simulink model "Simulation_wrapped_4"  (R2015a)
settings: Solver=ode4  SolverMode=SingleTasking  StartTime=0.0  StopTime=20  FixedStep=0.001  MaxStep=0.01  RelTol=1e-3
InitFcn:
  | gen_signal
  | Read_aero_spreadsheet
  | model_params3
undefined symbols (not defined in the file or in its folder): acm_aero_model, acm_pitch_deg_ini, acm_pitch_rate_deg_s_ini, acm_T_N, breakpoints1, Cm0, Cmde, Cmq, dail, de, dele, drud, Fr_mp_1, Fr_mp_2, Fr_rp_1, Fr_rp_2, ini_acm_de_deg, ini_acm_p_deg_per_s, ini_acm_phi_deg, ini_acm_psi_deg, ini_acm_q_deg_per_s, ini_acm_r_deg_per_s, ini_acm_theta_deg, ini_cmp_de_deg, ini_rig_p_deg_per_s, ini_rig_phi_deg, ini_rig_psi_deg, ini_rig_q_deg_per_s, ini_rig_r_deg_per_s, ini_rig_theta_deg, ini_rig_theta_deg_per_s, K1_svo_acm, K1_svo_cmp, K2_svo_acm, K2_svo_cmp, K_de_nz2, K_de_q2, K_de_tht2, La, Ma, max_defl_sat_acm, max_defl_sat_cmp, max_rate_sat, max_rate_sat_acm, max_rate_sat_cmp, Na, rig_pitch_deg_ini, rig_pitch_rate_deg_s_ini, sigbuilder_block, simstop, windspeed, Xa, Ya, Za
libraries: aerolibconvert2 x96, simulink x40, aerolibtransform2 x18, vrlib x7
(part 1 of 6)
settings Model: CovSFcnEnable=off  Creator=PD Banneheka  LastModifiedBy=PD Banneheka
settings DataIOCC: SignalLoggingSaveFormat=ModelDataLogs  ReturnWorkspaceOutputs=on
settings DebuggingCC: ReadBeforeWriteMsg=DisableAll  WriteAfterWriteMsg=DisableAll  WriteAfterReadMsg=DisableAll  AlgebraicLoopMsg=none  ArtificialAlgebraicLoopMsg=none  UnderspecifiedInitializationDetection=Classic  MergeDetectMultiDrivingBlocksExec=none  SolverPrmCheckMsg=warning  MultiTaskDSMMsg=warning  MultiTaskCondExecSysMsg=none  StateNameClashWarn=warning
settings HardwareCC: ProdBitPerInt=16  ProdBitPerPointer=16  ProdWordSize=16  ProdHWDeviceType=Generic->16-bit Embedded Processor
settings ModelReferenceCC: UpdateModelReferenceTargets=IfOutOfDate  ModelReferenceMinAlgLoopOccurrences=on
settings SFSimCC: SimUserIncludeDirs=D:\PhD\2016\Week_27_25_Apr\Matlab\Simulation_load_cell\HHIRM  SFSimEcho=off

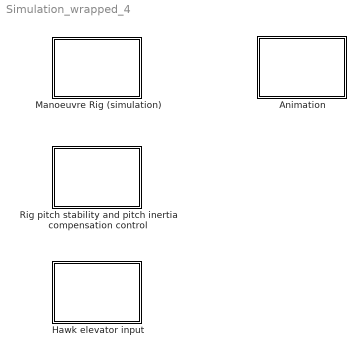
== system Simulation_wrapped_4 ==
  Animation : Subsystem
  Hawk elevator input : Subsystem
  Manoeuvre Rig (simulation) : Subsystem
  "Rig pitch stability and pitch inertia compensation control " : Subsystem

== system Simulation_wrapped_4/Animation ==
  Rotation Matrix to VRML Rotation{,1,3..6} (6 alike) : vrlib/Utilities/Rotation Matrix to VRML Rotation  maxzero=1e-12
  VR Sink : vrlib/VR Sink  InstantiateOnLoad=on  SampleTime=-1  ViewEnable=on  RemoteChange=off  RemoteView=off  FieldsWritten=Compensator.rotation.4.1.1.double#Compensator.translation.3.1.1.double#Arm.rotation.4.1.1.double#Arm.translation.3.1.1.double#Aircraft_model.rotation.4.1.1.double#Aircraft_model.translation.3.1.1.double#Back_added_mass.rotation.4.1.1.double#Back_added_mass.translation.3.1.1.double#Load_cell.rotation.4.1.1.double#Load_cell.translation.3.1.1.double#Link.rotation.4.1.1.double#Link.translation.3.1.1.double  WorldFileName=Animation.wrl  AutoView=on  VideoDimensions=[]  AllowVariableSize=off  FigureProperties="{'Position', 'Name', 'Viewpoint', 'CameraBound', 'CameraDirection', 'CameraPosition', 'CameraUpVector', 'ZoomFactor', 'Antialiasing', 'Headlight', 'Lighting', 'NavPanel', 'Sound', 'StatusBar', 'Stereo3D', 'Stereo3DCameraOffset', 'Stereo3DHIT', 'ToolBar', 'Textures', 'Transparency', 'Triad', 'Wireframe', 'NavZones', 'NavMode', 'NavSpeed', 'CaptureFileFormat', 'CaptureFileName', 'Record2DCompressMethod', 'Record2DCompressQuality', 'Record2D', 'Record2DFileName', 'Record2DFPS'; [1.9220000000000000e+03   8.4000000000000000e+01   9.5800000000000000e+02   3.8400000000000000e+02], '', 'Side view', 'on', [0.0000000000000000e+00   0.0000000000000000e+00  -1.0000000000000000e+00], [0.0000000000000000e+00   0.0000000000000000e+00   0.0000000000000000e+00], [0.0000000000000000e+00   1.0000000000000000e+00   0.0000000000000000e+00], [1.0000000000000000e+00], 'on', 'on', 'on', 'halfbar', 'on', 'on', 'off', [1.0000000149011612e-01], [0.0000000000000000e+00], 'on', 'on', 'on', 'none', 'off', 'off', 'fly', 'normal', 'tif', '%f_anim_%n.tif', 'auto', [7.5000000000000000e+01], 'off', '%f_anim_%n.avi', 'auto'}"
  wires:
  [animation_cmp_rotation] -> Rotation Matrix to VRML Rotation/1
  [animation_acm_rotation] -> Rotation Matrix to VRML Rotation4/1
  [animation_mass_rotation] -> Rotation Matrix to VRML Rotation3/1
  [animation_arm_rotation] -> Rotation Matrix to VRML Rotation1/1
  [animation_load_cell_rotation] -> Rotation Matrix to VRML Rotation5/1
  [animation_link_rotation] -> Rotation Matrix to VRML Rotation6/1
  [animation_link_translation] -> VR Sink/12
  Rotation Matrix to VRML Rotation/1 -> VR Sink/1
  [animation_cmp_translation] -> VR Sink/2
  Rotation Matrix to VRML Rotation1/1 -> VR Sink/3
  [animation_arm_translation] -> VR Sink/4
  Rotation Matrix to VRML Rotation4/1 -> VR Sink/5
  [animation_acm_translation] -> VR Sink/6
  Rotation Matrix to VRML Rotation3/1 -> VR Sink/7
  [animation_mass_translation] -> VR Sink/8
  Rotation Matrix to VRML Rotation5/1 -> VR Sink/9
  [animation_load_cell_translation] -> VR Sink/10
  Rotation Matrix to VRML Rotation6/1 -> VR Sink/11

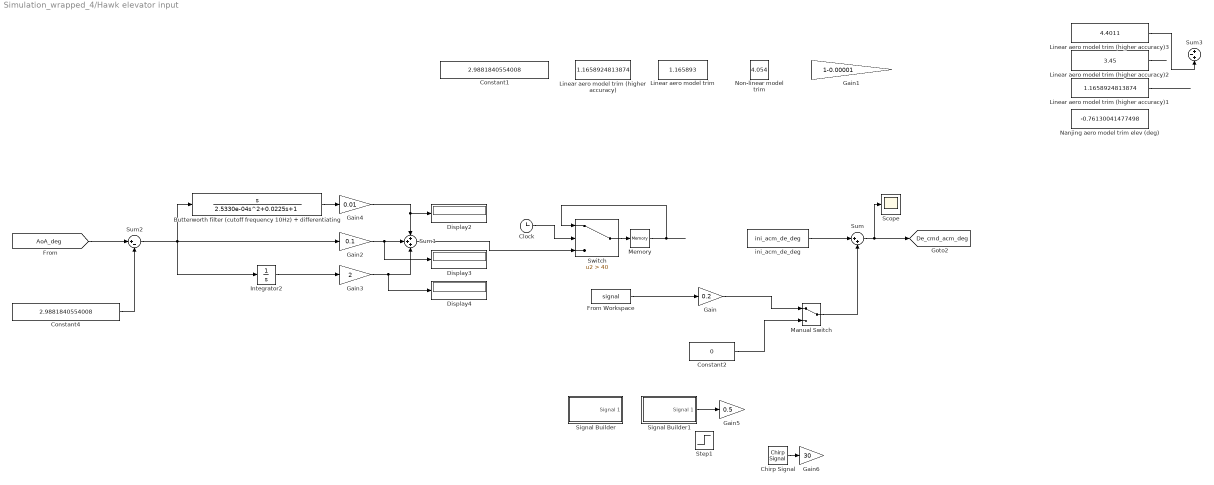
== system Simulation_wrapped_4/Hawk elevator input ==
  Butterworth filter (cutoff frequency 10Hz) + differentiating : TransferFcn  Numerator=[1 0]  Denominator=[2.5330e-04 0.0225 1]
  Chirp Signal : simulink/Sources/Chirp Signal  f1=0.1  T=100  f2=1
  Clock : Clock
  Constant1 : Constant  Value=2.9881840554008
  Constant2 : Constant  Value=0
  Constant4 : Constant  Value=2.9881840554008
  Display2 : Display
  Display3 : Display
  Display4 : Display
  From Workspace : FromWorkspace  VariableName=signal  SampleTime=0  OutputAfterFinalValue=Setting to zero
  Gain : Gain  Gain=0.2
  Gain1 : Gain  Gain=1-0.00001
  Gain2 : Gain  Gain=0.1
  Gain3 : Gain  Gain=2
  Gain4 : Gain  Gain=0.01
  Gain5 : Gain  Gain=0.5
  Gain6 : Gain  Gain=30
  Integrator2 : Integrator
  Linear aero model trim : Constant  Value=1.165893
  Linear aero model trim (higher accuracy) : Constant  Value=1.1658924813874
  Linear aero model trim (higher accuracy)1 : Constant  Value=1.1658924813874
  Linear aero model trim (higher accuracy)2 : Constant  Value=3.45
  Linear aero model trim (higher accuracy)3 : Constant  Value=4.4011
  Manual Switch : ManualSwitch
  Memory : Memory
  Nanjing aero model trim elev (deg) : Constant  Value=-0.76130041477498
  Non-linear model trim : Constant  Value=4.054
  Scope : Scope
      settings: SaveName=ScopeData7
  Signal Builder : Subsystem  Tag=STV Subsys  LoadFcn=sigbuilder_block('load');  StartFcn=sigbuilder_block('start');  StopFcn=sigbuilder_block('stop');  ClipboardFcn=sigbuilder_block('clipboard');  mask(Sigbuilder block){}
      mask help: Simulink:masks:SigbuilderBlock_MD
      mask init:
      | if ~strcmp(get_param(bdroot(gcbh),'SimulationStatus'),'stopped') tuvar = sigbuilder_block('maskInit'); end
      settings: CopyFcn=sigbuilder_block('copy');  DeleteFcn=sigbuilder_block('delete');  ModelCloseFcn=sigbuilder_block('modelClose');  PreSaveFcn=sigbuilder_block('preSave');  PauseFcn=sigbuilder_block('pause');  ContinueFcn=sigbuilder_block('continue');  NameChangeFcn=sigbuilder_block('namechange');  OpenFcn=sigbuilder_block('open',[437.6 199.2 550.4 400 ]);  CloseFcn=sigbuilder_block('close');
      mask Display: plot(0, 0, 100, 100,[2, 2, 32, 32, 2], [68, 8, 8, 68, 68],[32, 2], [38, 38], [32, 19, 2],[53, 60, 44], [32, 17, 17, 2],[16, 16, 31, 31]);txt = getActiveGroup(gcbh);text(2, 100, txt,'verticalAlignment', 'top');
  Signal Builder1 : Subsystem  Tag=STV Subsys  LoadFcn=sigbuilder_block('load');  StartFcn=sigbuilder_block('start');  StopFcn=sigbuilder_block('stop');  ClipboardFcn=sigbuilder_block('clipboard');  mask(Sigbuilder block){}
      mask help: Simulink:masks:SigbuilderBlock_MD
      mask init:
      | if ~strcmp(get_param(bdroot(gcbh),'SimulationStatus'),'stopped') tuvar = sigbuilder_block('maskInit'); end
      settings: CopyFcn=sigbuilder_block('copy');  DeleteFcn=sigbuilder_block('delete');  ModelCloseFcn=sigbuilder_block('modelClose');  PreSaveFcn=sigbuilder_block('preSave');  PauseFcn=sigbuilder_block('pause');  ContinueFcn=sigbuilder_block('continue');  NameChangeFcn=sigbuilder_block('namechange');  OpenFcn=sigbuilder_block('open',[437.6 199.2 550.4 400 ]);  CloseFcn=sigbuilder_block('close');
      mask Display: plot(0, 0, 100, 100,[2, 2, 32, 32, 2], [68, 8, 8, 68, 68],[32, 2], [38, 38], [32, 19, 2],[53, 60, 44], [32, 17, 17, 2],[16, 16, 31, 31]);txt = getActiveGroup(gcbh);text(2, 100, txt,'verticalAlignment', 'top');
  Step1 : Step  After=40-4.4011  SampleTime=0
  Sum : Sum  Inputs=|++
  Sum1 : Sum  Inputs=+++
  Sum2 : Sum  Inputs=|+-
  Sum3 : Sum  Inputs=+-+
  Switch : Switch  Criteria=u2 > Threshold  Threshold=40
  ini_acm_de_deg : Constant  Value=ini_acm_de_deg
  tag scope: De_cmd_acm_deg=global
  wires:
  From Workspace/1 -> Gain/1
  Manual Switch/1 -> Sum/2
  Gain/1 -> Manual Switch/1
  Integrator2/1 -> Gain3/1
  Sum2/1 -> Integrator2/1, Gain2/1, Butterworth filter (cutoff frequency 10Hz) + differentiating/1
  Butterworth filter (cutoff frequency 10Hz) + differentiating/1 -> Gain4/1
  Gain2/1 -> Display3/1, Sum1/2
  Gain4/1 -> Display2/1, Sum1/1
  Gain3/1 -> Display4/1, Sum1/3
  Sum1/1 -> Switch/3
  Switch/1 -> Memory/1
  Clock/1 -> Switch/2
  Memory/1 -> Switch/1
  [AoA_deg] -> Sum2/1
  Constant4/1 -> Sum2/2
  ini_acm_de_deg/1 -> Sum/1
  Signal Builder1/1(Signal 1) -> Gain5/1
  Sum/1 -> Scope/1, [De_cmd_acm_deg]
  Constant2/1 -> Manual Switch/2
  Chirp Signal/1 -> Gain6/1
  Linear aero model trim (higher accuracy)3/1 -> Sum3/3
  Linear aero model trim (higher accuracy)1/1 -> ?
  Linear aero model trim (higher accuracy)2/1 -> ?

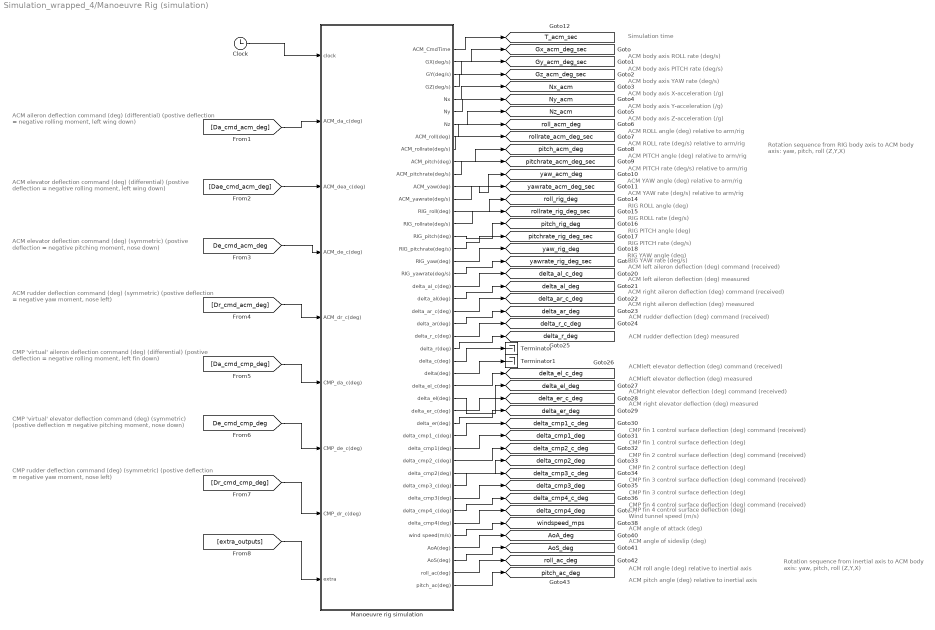
== system Simulation_wrapped_4/Manoeuvre Rig (simulation) ==
  note: ACM aileron deflection command (deg) (differential)
      | (postive deflection = negative rolling moment, left wing down)
  note: Wind tunnel speed (m/s)
  note: CMP fin 1 control surface deflection (deg) command (received)
  note: ACM left aileron deflection (deg) command (received)
  note: Simulation time
  note: ACM body axis ROLL rate (deg/s)
  note: ACM body axis PITCH rate (deg/s)
  note: ACM body axis YAW rate (deg/s)
  note: ACM body axis X-acceleration (/g)
  note: ACM body axis Y-acceleration (/g)
  note: ACM body axis Z-acceleration (/g)
  note: ACM ROLL angle (deg) relative to arm/rig
  note: ACM PITCH angle (deg) relative to arm/rig
  note: ACM YAW angle (deg) relative to arm/rig
  note: Rotation sequence from RIG body axis to ACM
      | body axis: yaw, pitch, roll (Z,Y,X)
  note: ACM ROLL rate (deg/s) relative to arm/rig
  note: ACM PITCH rate (deg/s) relative to arm/rig
  note: ACM YAW rate (deg/s) relative to arm/rig
  note: RIG ROLL angle (deg)
  note: RIG PITCH angle (deg)
  note: RIG YAW angle (deg)
  note: RIG ROLL rate (deg/s)
  note: RIG PITCH rate (deg/s)
  note: RIG YAW rate (deg/s)
  note: ACM left aileron deflection (deg) measured
  note: ACM right aileron deflection (deg) measured
  note: ACM right aileron deflection (deg) command (received)
  note: ACM rudder deflection (deg) measured
  note: ACM rudder deflection (deg) command (received)
  note: ACMleft elevator deflection (deg) measured
  note: ACMleft elevator deflection (deg) command (received)
  note: ACM right elevator deflection (deg) measured
  note: ACMright elevator deflection (deg) command (received)
  note: CMP fin 1 control surface deflection (deg)
  note: CMP fin 2 control surface deflection (deg) command (received)
  note: CMP fin 2 control surface deflection (deg)
  note: CMP fin 3 control surface deflection (deg) command (received)
  note: CMP fin 3 control surface deflection (deg)
  note: CMP fin 4 control surface deflection (deg) command (received)
  note: CMP fin 4 control surface deflection (deg)
  note: ACM angle of attack (deg)
  note: ACM angle of sideslip (deg)
  note: ACM roll angle (deg) relative to inertial axis
  note: ACM pitch angle (deg) relative to inertial axis
  note: Rotation sequence from inertial axis to ACM
      | body axis: yaw, pitch, roll (Z,Y,X)
  note: ACM elevator deflection command (deg) (symmetric)
      | (postive deflection = negative pitching moment, nose down)
  note: ACM rudder deflection command (deg) (symmetric)
      | (postive deflection = negative yaw moment, nose left)
  note: CMP 'virtual' aileron deflection command (deg) (differential)
      | (postive deflection = negative rolling moment, left fin down)
  note: CMP 'virtual' elevator deflection command (deg) (symmetric)
      | (postive deflection = negative pitching moment, nose down)
  note: CMP rudder deflection command (deg) (symmetric)
      | (postive deflection = negative yaw moment, nose left)
  note: ACM elevator deflection command (deg) (differential)
      | (postive deflection = negative rolling moment, left wing down)
  Clock : Clock
  Manoeuvre rig simulation : Subsystem
  Terminator : Terminator
  Terminator1 : Terminator
  tag scope: AoA_deg=global, AoS_deg=global, Gx_acm_deg_sec=global, Gy_acm_deg_sec=global, Gz_acm_deg_sec=global, Nx_acm=global, Ny_acm=global, Nz_acm=global, T_acm_sec=global, delta_al_c_deg=global, delta_al_deg=global, delta_ar_c_deg=global, delta_ar_deg=global, delta_cmp1_c_deg=global, delta_cmp1_deg=global, delta_cmp2_c_deg=global, delta_cmp2_deg=global, delta_cmp3_c_deg=global, delta_cmp3_deg=global, delta_cmp4_c_deg=global, delta_cmp4_deg=global, delta_el_c_deg=global, delta_el_deg=global, delta_er_c_deg=global, delta_er_deg=global, delta_r_c_deg=global, delta_r_deg=global, pitch_ac_deg=global, pitch_acm_deg=global, pitch_rig_deg=global, pitchrate_acm_deg_sec=global, pitchrate_rig_deg_sec=global, roll_ac_deg=global, roll_acm_deg=global, roll_rig_deg=global, rollrate_acm_deg_sec=global, rollrate_rig_deg_sec=global, windspeed_mps=global, yaw_acm_deg=global, yaw_rig_deg=global, yawrate_acm_deg_sec=global, yawrate_rig_deg_sec=global
  wires:
  Manoeuvre rig simulation/26(delta_c(deg)) -> Terminator/1
  Manoeuvre rig simulation/27(delta(deg)) -> Terminator1/1
  Manoeuvre rig simulation/1(ACM_CmdTime) -> [T_acm_sec]
  Manoeuvre rig simulation/2(GX(deg/s)) -> [Gx_acm_deg_sec]
  Manoeuvre rig simulation/3(GY(deg/s)) -> [Gy_acm_deg_sec]
  Manoeuvre rig simulation/4(GZ(deg/s)) -> [Gz_acm_deg_sec]
  Manoeuvre rig simulation/5(Nx) -> [Nx_acm]
  Manoeuvre rig simulation/6(Ny) -> [Ny_acm]
  Manoeuvre rig simulation/7(Nz) -> [Nz_acm]
  Manoeuvre rig simulation/8(ACM_roll(deg)) -> [roll_acm_deg]
  Manoeuvre rig simulation/9(ACM_rollrate(deg/s)) -> [rollrate_acm_deg_sec]
  Manoeuvre rig simulation/10(ACM_pitch(deg)) -> [pitch_acm_deg]
  Manoeuvre rig simulation/11(ACM_pitchrate(deg/s)) -> [pitchrate_acm_deg_sec]
  Manoeuvre rig simulation/12(ACM_yaw(deg)) -> [yaw_acm_deg]
  Manoeuvre rig simulation/13(ACM_yawrate(deg/s)) -> [yawrate_acm_deg_sec]
  Manoeuvre rig simulation/14(RIG_roll(deg)) -> [roll_rig_deg]
  Manoeuvre rig simulation/15(RIG_rollrate(deg/s)) -> [rollrate_rig_deg_sec]
  Manoeuvre rig simulation/16(RIG_pitch(deg)) -> [pitch_rig_deg]
  Manoeuvre rig simulation/17(RIG_pitchrate(deg/s)) -> [pitchrate_rig_deg_sec]
  Manoeuvre rig simulation/18(RIG_yaw(deg)) -> [yaw_rig_deg]
  Manoeuvre rig simulation/19(RIG_yawrate(deg/s)) -> [yawrate_rig_deg_sec]
  Manoeuvre rig simulation/20(delta_al_c(deg)) -> [delta_al_c_deg]
  Manoeuvre rig simulation/21(delta_al(deg)) -> [delta_al_deg]
  Manoeuvre rig simulation/22(delta_ar_c(deg)) -> [delta_ar_c_deg]
  Manoeuvre rig simulation/23(delta_ar(deg)) -> [delta_ar_deg]
  Manoeuvre rig simulation/24(delta_r_c(deg)) -> [delta_r_c_deg]
  Manoeuvre rig simulation/25(delta_r(deg)) -> [delta_r_deg]
  Manoeuvre rig simulation/28(delta_el_c(deg)) -> [delta_el_c_deg]
  Manoeuvre rig simulation/29(delta_el(deg)) -> [delta_el_deg]
  Manoeuvre rig simulation/30(delta_er_c(deg)) -> [delta_er_c_deg]
  Manoeuvre rig simulation/31(delta_er(deg)) -> [delta_er_deg]
  Manoeuvre rig simulation/32(delta_cmp1_c(deg)) -> [delta_cmp1_c_deg]
  Manoeuvre rig simulation/33(delta_cmp1(deg)) -> [delta_cmp1_deg]
  Manoeuvre rig simulation/34(delta_cmp2_c(deg)) -> [delta_cmp2_c_deg]
  Manoeuvre rig simulation/35(delta_cmp2(deg)) -> [delta_cmp2_deg]
  Manoeuvre rig simulation/36(delta_cmp3_c(deg)) -> [delta_cmp3_c_deg]
  Manoeuvre rig simulation/37(delta_cmp3(deg)) -> [delta_cmp3_deg]
  Manoeuvre rig simulation/38(delta_cmp4_c(deg)) -> [delta_cmp4_c_deg]
  Manoeuvre rig simulation/39(delta_cmp4(deg)) -> [delta_cmp4_deg]
  Manoeuvre rig simulation/41(AoA(deg)) -> [AoA_deg]
  Manoeuvre rig simulation/42(AoS(deg)) -> [AoS_deg]
  Manoeuvre rig simulation/43(roll_ac(deg)) -> [roll_ac_deg]
  Manoeuvre rig simulation/44(pitch_ac(deg)) -> [pitch_ac_deg]
  Manoeuvre rig simulation/40(wind speed(m/s)) -> [windspeed_mps]
  [extra_outputs] -> Manoeuvre rig simulation/9(extra)
  [Da_cmd_acm_deg] -> Manoeuvre rig simulation/2(ACM_da_c(deg))
  [Dae_cmd_acm_deg] -> Manoeuvre rig simulation/3(ACM_dea_c(deg))
  [De_cmd_acm_deg] -> Manoeuvre rig simulation/4(ACM_de_c(deg))
  [Dr_cmd_acm_deg] -> Manoeuvre rig simulation/5(ACM_dr_c(deg))
  [Da_cmd_cmp_deg] -> Manoeuvre rig simulation/6(CMP_da_c(deg))
  [De_cmd_cmp_deg] -> Manoeuvre rig simulation/7(CMP_de_c(deg))
  [Dr_cmd_cmp_deg] -> Manoeuvre rig simulation/8(CMP_dr_c(deg))
  Clock/1 -> Manoeuvre rig simulation/1(clock)

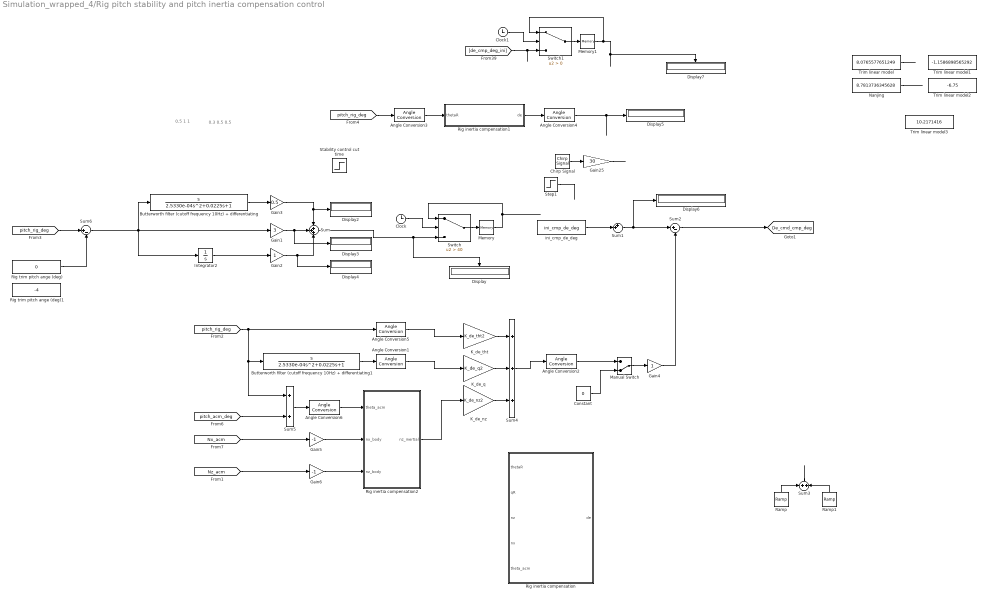
== system Simulation_wrapped_4/Rig pitch stability and pitch inertia compensation control  ==
  note: 0.3
      | 0.5
      | 0.5
  note: 0.5
      | 1
      | 1
  Angle Conversion{1,3,5..6} (4 alike) : aerolibconvert2/Angle Conversion  IU=deg  OU=rad
  Angle Conversion2 : aerolibconvert2/Angle Conversion  IU=rad  OU=deg
  Angle Conversion4 : aerolibconvert2/Angle Conversion  IU=rad  OU=deg
  Butterworth filter (cutoff frequency 10Hz) + differentiating : TransferFcn  Numerator=[1 0]  Denominator=[2.5330e-04 0.0225 1]
  Butterworth filter (cutoff frequency 10Hz) + differentiating1 : TransferFcn  Numerator=[1 0]  Denominator=[2.5330e-04 0.0225 1]
  Chirp Signal : simulink/Sources/Chirp Signal  f1=0.3  T=600  f2=1.0
  Clock : Clock
  Clock1 : Clock
  Constant : Constant  Value=0
  Display{,2..7} (7 alike) : Display
  Gain1 : Gain  Gain=3
  Gain2 : Gain
  Gain25 : Gain  Gain=30
  Gain3 : Gain  Gain=0.5
  Gain4 : Gain
  Gain5 : Gain  Gain=-1
  Gain6 : Gain  Gain=-1
  Integrator2 : Integrator
  K_de_nz : Gain  Gain=K_de_nz2
  K_de_q : Gain  Gain=K_de_q2
  K_de_tht : Gain  Gain=K_de_tht2
  Manual Switch : ManualSwitch  CurrentSetting=0
  Memory : Memory
  Memory1 : Memory
  Nanjing : Constant  Value=8.7813736345628
  Ramp : simulink/Sources/Ramp  slope=1/10  start=10  X0=0
  Ramp1 : simulink/Sources/Ramp  slope=-1/10  start=20  X0=0
  Rig inertia compensation : MATLAB Function  TreatAsAtomicUnit=on
  Rig inertia compensation1 : MATLAB Function  TreatAsAtomicUnit=on
  Rig inertia compensation2 : MATLAB Function  TreatAsAtomicUnit=on
  Rig trim pitch ange (deg) : Constant  Value=0
  Rig trim pitch ange (deg)1 : Constant  Value=-4
  Stability control cut time : Step  Time=40  Before=1  After=0  SampleTime=0
  Step1 : Step  After=-40-10.21714  SampleTime=0
  Sum : Sum  Inputs=+++
  Sum1 : Sum  Inputs=++|
  Sum2 : Sum  Inputs=|+-
  Sum3 : Sum
  Sum4 : Sum  Inputs=+++
  Sum5 : Sum
  Sum6 : Sum  Inputs=|+-
  Switch : Switch  Criteria=u2 > Threshold  Threshold=40
  Switch1 : Switch  Criteria=u2 > Threshold
  Trim linear model : Constant  Value=8.0765577651249
  Trim linear model1 : Constant  Value=-1.1586898565292
  Trim linear model2 : Constant  Value=-6.75
  Trim linear model3 : Constant  Value=10.2171416
  ini_cmp_de_deg : Constant  Value=ini_cmp_de_deg
  tag scope: De_cmd_cmp_deg=global
  wires:
  Integrator2/1 -> Gain2/1
  Sum6/1 -> Integrator2/1, Gain1/1, Butterworth filter (cutoff frequency 10Hz) + differentiating/1
  Butterworth filter (cutoff frequency 10Hz) + differentiating/1 -> Gain3/1
  Gain1/1 -> Display3/1, Sum/2
  Gain3/1 -> Display2/1, Sum/1
  Gain2/1 -> Display4/1, Sum/3
  Butterworth filter (cutoff frequency 10Hz) + differentiating1/1 -> Angle Conversion1/1
  Ramp1/1 -> Sum3/2
  Ramp/1 -> Sum3/1
  Sum3/1 -> ?
  Switch/1 -> Memory/1
  Angle Conversion2/1 -> Manual Switch/1
  Constant/1 -> Manual Switch/2
  Manual Switch/1 -> Gain4/1
  Sum1/1 -> Display6/1, Sum2/1
  Gain4/1 -> Sum2/2
  Angle Conversion3/1 -> Rig inertia compensation1/1(thetaR)
  [pitch_rig_deg] -> Angle Conversion3/1
  Rig inertia compensation1/1(de) -> Angle Conversion4/1
  Angle Conversion4/1 -> Display5/1
  [Nx_acm] -> Gain5/1
  Clock/1 -> Switch/2
  Sum/1 -> Display/1, Switch/3
  Angle Conversion1/1 -> K_de_q/1
  K_de_tht/1 -> Sum4/1
  K_de_q/1 -> Sum4/2
  K_de_nz/1 -> Sum4/3
  Angle Conversion5/1 -> K_de_tht/1
  Sum4/1 -> Angle Conversion2/1
  Gain5/1 -> Rig inertia compensation2/2(nx_body)
  [pitch_rig_deg] -> Angle Conversion5/1, Butterworth filter (cutoff frequency 10Hz) + differentiating1/1, Sum5/1
  [pitch_acm_deg] -> Sum5/2
  Sum5/1 -> Angle Conversion6/1
  Angle Conversion6/1 -> Rig inertia compensation2/1(theta_acm)
  [Nz_acm] -> Gain6/1
  Rig inertia compensation2/1(nz_inertial) -> K_de_nz/1
  Gain6/1 -> Rig inertia compensation2/3(nz_body)
  Memory/1 -> Switch/1
  Switch1/1 -> Memory1/1
  Clock1/1 -> Switch1/2
  [de_cmp_deg_ini] -> Switch1/3
  Memory1/1 -> Display7/1, Switch1/1
  Sum2/1 -> [De_cmd_cmp_deg]
  [pitch_rig_deg] -> Sum6/1
  Rig trim pitch ange (deg)/1 -> Sum6/2
  ini_cmp_de_deg/1 -> Sum1/2
  Step1/1 -> ?
  Trim linear model/1 -> ?
  Nanjing/1 -> ?
  Chirp Signal/1 -> Gain25/1
  Gain25/1 -> ?

== system Simulation_wrapped_4/Hawk elevator input/Signal Builder ==
  Demux : Demux  Tag=STV Demux  Outputs=1
  FromWs : FromWorkspace  Tag=STV FromWs  VariableName=tuvar  SampleTime=0
      SigBuilderData=|
      | common.afterFinalStr = 'Extrapolate'
      | common.sampleTime = 0
      | dataSet.timeRange = [0 10]
      | dataSet.name = 'Group 1'
      | sbobj.Groups.Name = 'Group 1'
      | sbobj.Groups.Signals.Name = 'Signal 1'
      | sbobj.Groups.Signals.XData = [0 2 2 3 3 4 4 10]
      | sbobj.Groups.Signals.YData = [0 0 -5 -5 5 5 0 0]
  Signal 1 : Outport  Tag=STV Outport
  wires:
  Demux/1 -> Signal 1/1
  FromWs/1 -> Demux/1

== system Simulation_wrapped_4/Hawk elevator input/Signal Builder1 ==
  Demux : Demux  Tag=STV Demux  Outputs=1
  FromWs : FromWorkspace  Tag=STV FromWs  VariableName=tuvar  SampleTime=0
      SigBuilderData=|
      | common.afterFinalStr = 'Extrapolate'
      | common.sampleTime = 0
      | dataSet.timeRange = [0 10]
      | dataSet.name = 'Group 1'
      | sbobj.Groups.Name = 'Group 1'
      | sbobj.Groups.Signals.Name = 'Signal 1'
      | sbobj.Groups.Signals.XData = [0 1 1 1.5 1.5 2 2 10]
      | sbobj.Groups.Signals.YData = [0 0 -40 -40 40 40 0 0]
  Signal 1 : Outport  Tag=STV Outport
  wires:
  FromWs/1 -> Demux/1
  Demux/1 -> Signal 1/1
